simulink subsystem "Battery"  (R2025b)
settings: Solver=VariableStepAuto  StartTime=0.0  StopTime=10.0  RelTol=1e-3
undefined symbols (not defined in the file): PlntBattCapInit, PlntBattChrgMax, PlntBattNumCellSer, PlntBattOpenCirctVolt, PlntBattVoltSocBpt
libraries: autolibdatasheetbattery x1
settings Model: ModifiedByFormat=The MathWorks, Inc.  Creator=The MathWorks, Inc.  LastModifiedBy=The MathWorks, Inc.
settings SolverCC: MaxZcPerStep=1.0
settings OptimizationCC: ReuseModelBlockBuffer=off
settings DebuggingCC: UnconnectedInputMsg=warning  UnconnectedOutputMsg=warning  UnconnectedLineMsg=warning
settings ModelReferenceCC: EnableRefExpFcnMdlSchedulingChecks=on
settings RTWCC: GPUComputeCapability=3.5  DLArmComputeVersion=19.05

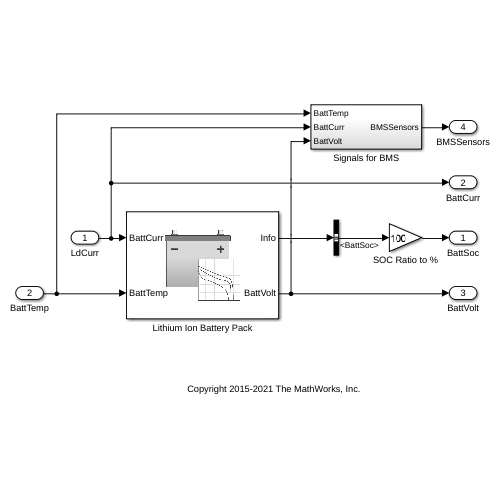
[thumbnail: Simulink's stored preview of the top-level diagram]
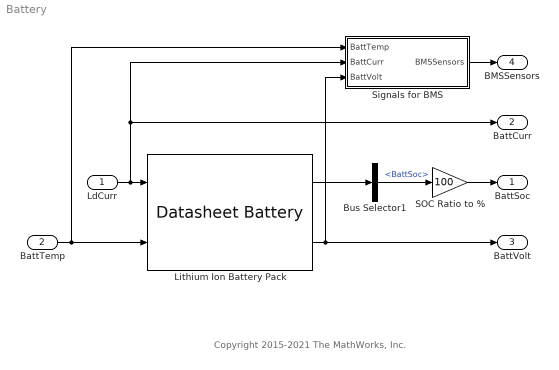
== system Battery ==
  note: Copyright 2015-2021 The MathWorks, Inc.
  LdCurr : Inport
  BattTemp : Inport  Port=2
  Bus Selector1 : BusSelector  OutputSignals=BattSoc
  Lithium Ion Battery Pack : autolibdatasheetbattery/Datasheet Battery  CapacityCtrl=Parameter  OutputVlt=Filtered  BattChargeMax=PlntBattChrgMax  Em=PlntBattOpenCirctVolt  SOCEmBp=PlntBattVoltSocBpt  RInt=PlntBattIntrnRes  BattTempBp=PlntBattTempBpt  SOCRintBp=PlntBattSocBpt  Ns=PlntBattNumCellSer  Np=PlntBattNumCellPar  BattCapInit=PlntBattCapInit  Tc=PlntBattTimeCnst  Vinit=PlntBattNumCellSer*interp1(PlntBattVoltSocBpt, PlntBattOpenCirctVolt, PlntBattCapInit/PlntBattChrgMax)  RefBlkName='autolibdatasheetbattery/Datasheet Battery'
  SOC Ratio to % : Gain  Gain=100
  Signals for BMS : Subsystem
  BattSoc : Outport  VectorParamsAs1DForOutWhenUnconnected=off
  BattCurr : Outport  Port=2  VectorParamsAs1DForOutWhenUnconnected=off
  BattVolt : Outport  Port=3  VectorParamsAs1DForOutWhenUnconnected=off
  BMSSensors : Outport  Port=4  VectorParamsAs1DForOutWhenUnconnected=off
  wires:
  Lithium Ion Battery Pack/2 -> Signals for BMS/3(BattVolt), BattVolt/1
  BattTemp/1 -> Signals for BMS/1(BattTemp), Lithium Ion Battery Pack/2
  Bus Selector1/1 -> SOC Ratio to %/1  "<BattSoc>"
  LdCurr/1 -> Signals for BMS/2(BattCurr), BattCurr/1, Lithium Ion Battery Pack/1
  SOC Ratio to %/1 -> BattSoc/1
  Lithium Ion Battery Pack/1 -> Bus Selector1/1
  Signals for BMS/1(BMSSensors) -> BMSSensors/1

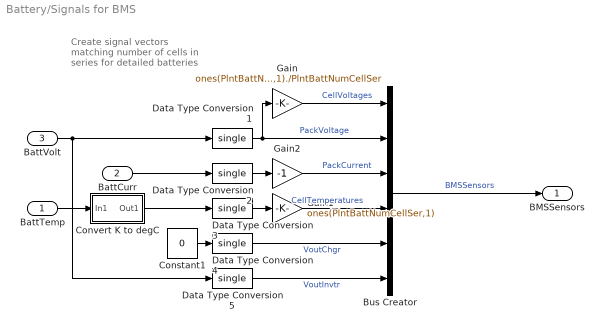
== system Battery/Signals for BMS ==
  note: Create signal vectors
      | matching number of
      | cells in series for
      | detailed batteries
  BattTemp : Inport
  BattCurr : Inport  Port=2
  BattVolt : Inport  Port=3
  Bus Creator : BusCreator  Inputs=6
  Constant1 : Constant  Value=0
  Convert K to degC : Subsystem
  Data Type Conversion{1..5} (5 alike) : DataTypeConversion  OutDataTypeStr=single  SaturateOnIntegerOverflow=off  RndMeth=Floor
  Gain : Gain  Gain=ones(PlntBattNumCellSer,1)./PlntBattNumCellSer
  Gain1 : Gain  Gain=ones(PlntBattNumCellSer,1)
  Gain2 : Gain  Gain=-1
  BMSSensors : Outport
  wires:
  Data Type Conversion2/1 -> Gain2/1
  Constant1/1 -> Data Type Conversion4/1
  Data Type Conversion1/1 -> Gain/1, Bus Creator/2  "PackVoltage"
  Gain/1 -> Bus Creator/1  "CellVoltages"
  BattVolt/1 -> Data Type Conversion5/1, Data Type Conversion1/1
  BattCurr/1 -> Data Type Conversion2/1
  BattTemp/1 -> Convert K to degC/1(In1)
  Convert K to degC/1(Out1) -> Data Type Conversion3/1
  Data Type Conversion4/1 -> Bus Creator/5  "VoutChgr"
  Gain1/1 -> Bus Creator/4  "CellTemperatures"
  Data Type Conversion5/1 -> Bus Creator/6  "VoutInvtr"
  Gain2/1 -> Bus Creator/3  "PackCurrent"
  Data Type Conversion3/1 -> Gain1/1
  Bus Creator/1 -> BMSSensors/1  "BMSSensors"

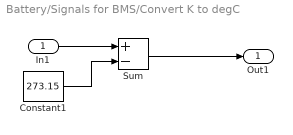
== system Battery/Signals for BMS/Convert K to degC ==
  In1 : Inport
  Constant1 : Constant  Value=273.15
  Sum : Sum  Inputs=+-
  Out1 : Outport
  wires:
  Sum/1 -> Out1/1
  Constant1/1 -> Sum/2
  In1/1 -> Sum/1
